simulink model "unifi_GFM_control_demo_single_conv"  (R2020b)
settings: Solver=VariableStepAuto  StartTime=0.0  StopTime=1  MaxStep=1e-3  RelTol=1e-3
InitFcn:
  | % VSC Rating
  | Vnomrms          = 120.0;                                              % [V]
  | Vnom               = Vnomrms*sqrt(2);                             % [V]
  | fnom                = 60.0;                                                % [Hz]
  | Wnom              = 2.0*pi*fnom;                                     % [rad/s]
  | Prated              = 3.0e3;                                               % [W]
  | Qrated             = 1.5e3;                                               % [VAR]
  | Inom               = 2.0*Prated/Vnom/3;                           % [A]
  | Zbase              = Vnom/Inom;                                      % [Ohm]
  | Lbase              = Zbase/Wnom;                                    % [H]
  | 
  | % LCL Filter parameters
  | L1                   = 600e-6;                                            % [H]
  | L2                   = 1e-3;                                                % [H]
  | Cf                    = 22e-6;                                              % [F]
  | R1                   = 20e-3;                                              % [Ohm]
  | R2                   = 20e-3;                                              % [Ohm]
  | Rf                    = 1.5;%20e-3;                                              % [Ohm]
  | 
  | % DC Bus
  | Vdc                  = 380.0;                                               % [V]
  | 
  | % Grid Parameters
  | xOverR             = 20.0;                                                 % [ratio]
  | Lg                    = Lbase*0.2;                                         % [H]
  | Rg                    = Zbase/xOverR*0.2                              % [Ohm]
  | 
  | 
  | % Firmware Parameters
  | IH                     = Inom*1.95;                                        % [A] - HW overcurrent trip limit (instantaneous value)
  | DCL                   = 2.0*Vnom/1.15*0.8;                           % [V]
  | DCH                  = Vdc*1.35;                                          % [V]
  | VGH                  = Vnom*1.5;                                         % [V]
  | 
  | % Droop Parameters
  | maxVolDev         = Vnom*0.05;                                       %[V]
  | maxFreqDev       = Wnom*0.01;                                      %[rad/s]
  | pwDroopCoeff     = maxFreqDev/Prated;                           %[rad/j]
  | qvDroopCoeff      = maxVolDev/Qrated;                            % [V/VAR]
StopFcn:
  | clear functions
libraries: powerlib x27, simulink x4, powerlib_meascontrol x2
settings Model: Creator=mawal  LastModifiedBy=mawal
settings SFSimCC: SimParseCustomCode=off  CustomCodeGlobalsAsFunctionIO=on

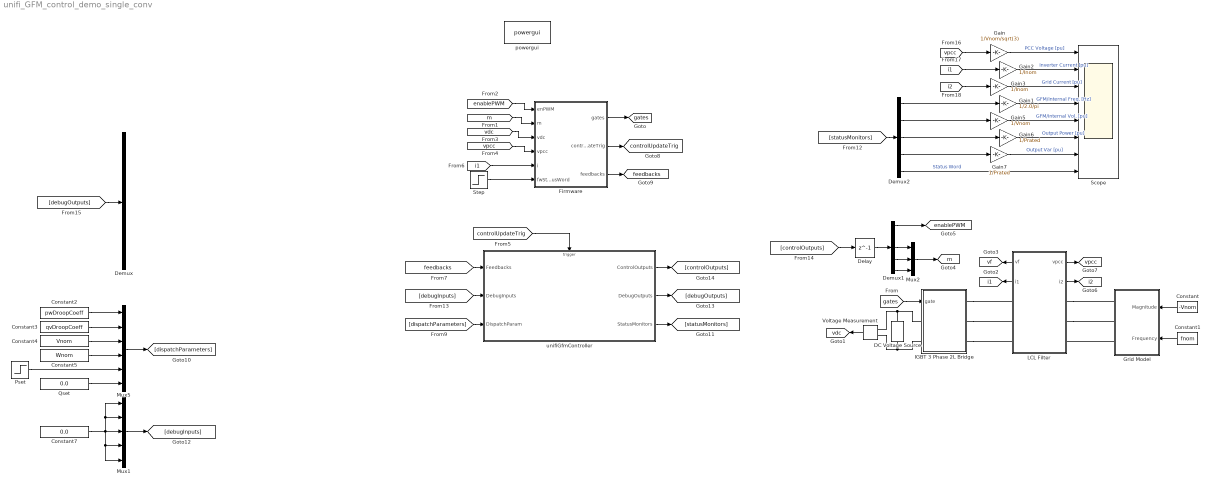
== system unifi_GFM_control_demo_single_conv ==
  Constant : Constant  Value=-Vnom  VectorParams1D=off  SampleTime=-1
  Constant1 : Constant  Value=fnom  VectorParams1D=off  SampleTime=-1
  Constant2 : Constant  Value=pwDroopCoeff
  Constant3 : Constant  Value=qvDroopCoeff
  Constant4 : Constant  Value=Vnom
  Constant5 : Constant  Value=Wnom
  Constant7 : Constant  Value=0.0
  DC Voltage Source : powerlib/Electrical Sources/DC Voltage Source  Amplitude=Vdc  Measurements=None
  Delay : Delay  DelayLength=1
  Demux : Demux  Outputs=10
  Demux1 : Demux  Outputs=5
  Demux2 : Demux  Outputs=5
  Firmware : Subsystem  mask{fsw=50e3, fs=25e3}
      mask prompts: fsw "Switching frequency"; fs "Sampling frequency"
  Gain : Gain  Gain=1/Vnom/sqrt(3)
  Gain1 : Gain  Gain=1/2.0/pi
  Gain2 : Gain  Gain=1/Inom
  Gain3 : Gain  Gain=1/Inom
  Gain5 : Gain  Gain=1/Vnom
  Gain6 : Gain  Gain=1/Prated
  Gain7 : Gain  Gain=1/Prated
  Grid Model : Subsystem
      settings: PortSchema="{\"entries\":[{\"content\":{\"sides\":[{\"content\":{\"connectorIds\":[\"LConn1\",\"LConn2\",\"LConn3\"]},\"type\":\"ConnectorPlacement.EquallySpacedRectSide\",\"uuid\":\"eac9bd49-6506-4418-b391-2d1910dfb123\"},{\"content\":{\"connectorIds\":[\"In1\",\"In2\"],\"side\":\"RIGHT\"},\"type\":\"ConnectorPlacement.EquallySpacedRectSide\",\"uuid\":\"2cf1b579-036f-4489-9916-029144d18b5e\"},{\"content\":{\"connectorIds\":[],\"side\":\"TOP\"},\"type\":\"ConnectorPlacement.EquallySpacedRectSide\",\"uuid\":\"45a6a27e-4276-40c1-8aac-6c9155e67f41\"},{\"content\":{\"connectorIds\":[],\"side\":\"BOTTOM\"},\"type\":\"ConnectorPlacement.EquallySpacedRectSide\",\"uuid\":\"f7ca4a45-1b00-4589-b172-9f3561ecadf3\"},{\"content\":{\"connectorIds\":[],\"side\":\"HIDDEN\"},\"type\":\"ConnectorPlacement.EquallySpacedRectSide\",\"uuid\":\"bf2ee3e7-e909-4e31-bcbb-76e709a5babf\"}]},\"type\":\"ConnectorPlacement.EquallySpacedConnector\",\"uuid\":\"022258a7-3899-4adf-8963-8d60febbe7fe\"}],\"packageUris\":[\"http://schema.mathworks.com/mf0/Connector/R2020b\"],\"version\":\"1.0\"}"
  IGBT 3 Phase 2L Bridge : Subsystem
  LCL Filter : Subsystem
      settings: PortSchema="{\"entries\":[{\"content\":{\"sides\":[{\"content\":{\"connectorIds\":[\"Out3\",\"Out4\",\"LConn1\",\"LConn2\",\"LConn3\"]},\"type\":\"ConnectorPlacement.EquallySpacedRectSide\",\"uuid\":\"3cdc7e29-4b8c-4f58-9b04-3ab9d7132857\"},{\"content\":{\"connectorIds\":[\"Out1\",\"Out2\",\"RConn1\",\"RConn2\",\"RConn3\"],\"side\":\"RIGHT\"},\"type\":\"ConnectorPlacement.EquallySpacedRectSide\",\"uuid\":\"8baa2de2-ce0c-48ae-b26c-b1033ca488ed\"},{\"content\":{\"connectorIds\":[],\"side\":\"TOP\"},\"type\":\"ConnectorPlacement.EquallySpacedRectSide\",\"uuid\":\"794c2f77-a18f-4e85-a713-f814f7818158\"},{\"content\":{\"connectorIds\":[],\"side\":\"HIDDEN\"},\"type\":\"ConnectorPlacement.EquallySpacedRectSide\",\"uuid\":\"a095602e-d5a6-4d5a-a12d-1bc7b692edfa\"}]},\"type\":\"ConnectorPlacement.EquallySpacedConnector\",\"uuid\":\"f071d9f2-7780-45fd-ac97-fd335e4ea6fb\"}],\"packageUris\":[\"http://schema.mathworks.com/mf0/Connector/R2020b\"],\"version\":\"1.0\"}"
  Mux1 : Mux  Inputs=5
  Mux2 : Mux  Inputs=3
  Mux5 : Mux  Inputs=6
  Pset : Step  Time=0.5  Before=0.0  After=Prated  SampleTime=0
  Qset : Constant  Value=0.0
  Scope : Scope  NumInputPorts=8
  Step : Step  Time=0  SampleTime=0
  Voltage Measurement : powerlib/Measurements/Voltage Measurement  PhasorSimulation=off  OutputType=Complex  PSBequivalent=0
  powergui : powerlib/powergui  Priority=1  SimulationMode=Continuous  SampleTime=0.2e-6  frequency=60  Iterations=50  frequencyindice=0  Pbase=100e6  ErrMax=1e-4  UnitsV=kV  UnitsW=MW  buscounter=0  FunctionMessages=off  echomessages=off  EnableUseOfTLC=off  CurrentSourceSwitches=off  DisableSnubberDevices=off  DisableRonSwitches=off  DisableVfSwitches=off  DisplayEquations=off  AutomaticDiscreteSolvers=off  SolverType=Tustin/Backward Euler (TBE)  Interpol=off  ExternalGateDelay=off  methode=off  Ts=100  x0status=blocks  SPID=on  SwTol=0  HookPort=off  NonlinearTolerance=1e-4  nMaxIteration=100  ContinueOnMaxIteration=off  RestoreLinks=warning  ResistiveCurrentMeasurement=off  Frange=[0:2:500]  Ylog=off  Xlog=on  ShowGrid=off  save=off  variable=ZData  structure=0  ZoomFFT=off  StartTime=0.0  cycles=1  DisplayStyle=1  fundamental=60  FreqAxis=off  MaxFrequency=1000  frequencyindicesteady=1  RmsSteady=1  display=off
  unifiGfmController : Subsystem  AncestorBlock=unifi_Sil_Lib/UNIFI SIL Wrapper with Mex Builder  TreatAsAtomicUnit=on
      mask DialogControl importSilTemplate Prompt: Step 1: Import SIL Template
      mask DialogControl importSilTemplate Callback: cbk_import_sil_tem
      mask DialogControl updateInterfaceDim Prompt: Step 2: Update Interface Dimensions (Add/Link custom code prior to Step 2)
      mask DialogControl updateInterfaceDim Callback: cbk_update_interface_dim
      mask DialogControl configMexBuilder Prompt: Step 3: Configure Mex Builder (Disable Library Link to Enable Self-Modification)
      mask DialogControl configMexBuilder Callback: cbk_setup_mex_builder
      mask DialogControl buildMex Prompt: Step 4: Build Mex
      mask DialogControl buildMex Callback: cbk_build_mex
      mask Display: image('$imagefile'); % Use "Edit Image" on toolstrip to change.
  tag scope: controlUpdateTrig=global, enablePWM=global, feedbacks=global, gates=global, i1=global, i2=global, m=global, vdc=global, vf=global, vpcc=global
  wires:
  unifiGfmController/2(DebugOutputs) -> [debugOutputs]
  Firmware/1(gates) -> [gates]
  [gates] -> IGBT 3 Phase 2L Bridge/1(gate)
  Voltage Measurement/1 -> [vdc]
  Constant/1 -> Grid Model/1(Magnitude)
  Constant1/1 -> Grid Model/2(Frequency)
  Demux1/3 -> Mux2/1
  Demux1/4 -> Mux2/2
  Demux1/5 -> Mux2/3
  Mux2/1 -> [m]
  Demux1/1 -> [enablePWM]
  [enablePWM] -> Firmware/1(enPWM)
  [m] -> Firmware/2(m)
  [vdc] -> Firmware/3(vdc)
  [vpcc] -> Firmware/4(vpcc)
  LCL Filter/4(i1) -> [i1]
  LCL Filter/3(vf) -> [vf]
  LCL Filter/2(i2) -> [i2]
  LCL Filter/1(vpcc) -> [vpcc]
  [i1] -> Firmware/5(i)
  Firmware/2(controlUpdateTrig) -> [controlUpdateTrig]
  Firmware/3(feedbacks) -> [feedbacks]
  [feedbacks] -> unifiGfmController/1(Feedbacks)
  Delay/1 -> Demux1/1
  Step/1 -> Firmware/6(fwStatusWord)
  Constant2/1 -> Mux5/1
  Constant3/1 -> Mux5/2
  Constant4/1 -> Mux5/3
  Constant5/1 -> Mux5/4
  Qset/1 -> Mux5/6
  Pset/1 -> Mux5/5
  [dispatchParameters] -> unifiGfmController/3(DispatchParam)
  Mux5/1 -> [dispatchParameters]
  unifiGfmController/3(StatusMonitors) -> [statusMonitors]
  [statusMonitors] -> Demux2/1
  Constant7/1 -> Mux1/2, Mux1/1, Mux1/3, Mux1/5, Mux1/4
  [debugInputs] -> unifiGfmController/2(DebugInputs)
  Mux1/1 -> [debugInputs]
  unifiGfmController/1(ControlOutputs) -> [controlOutputs]
  [controlOutputs] -> Delay/1
  [debugOutputs] -> Demux/1
  Demux2/5 -> Scope/8  "Status Word"
  Demux2/4 -> Gain7/1
  Demux2/3 -> Gain6/1
  Demux2/1 -> Gain1/1
  [vpcc] -> Gain/1
  Gain/1 -> Scope/1  "PCC Voltage [pu]"
  [i1] -> Gain2/1
  Gain2/1 -> Scope/2  "Inverter Current [pu]"
  [i2] -> Gain3/1
  Gain3/1 -> Scope/3  "Grid Current [pu]"
  Gain1/1 -> Scope/4  "GFM/Internal Freq. [Hz]"
  Demux2/2 -> Gain5/1
  Gain5/1 -> Scope/5  "GFM/Internal Vol. [pu]"
  Gain6/1 -> Scope/6  "Output Power [pu]"
  Gain7/1 -> Scope/7  "Output Var [pu]"
  [controlUpdateTrig] -> unifiGfmController/Trigger
  connections:
  IGBT 3 Phase 2L Bridge/RConn2 -- LCL Filter/LConn2
  IGBT 3 Phase 2L Bridge/RConn1 -- LCL Filter/LConn1
  IGBT 3 Phase 2L Bridge/RConn3 -- LCL Filter/LConn3
  DC Voltage Source/RConn1 -- Voltage Measurement/LConn1 -- IGBT 3 Phase 2L Bridge/LConn1
  DC Voltage Source/LConn1 -- Voltage Measurement/LConn2 -- IGBT 3 Phase 2L Bridge/LConn2
  LCL Filter/RConn1 -- Grid Model/LConn1
  LCL Filter/RConn2 -- Grid Model/LConn2
  Grid Model/LConn3 -- LCL Filter/RConn3

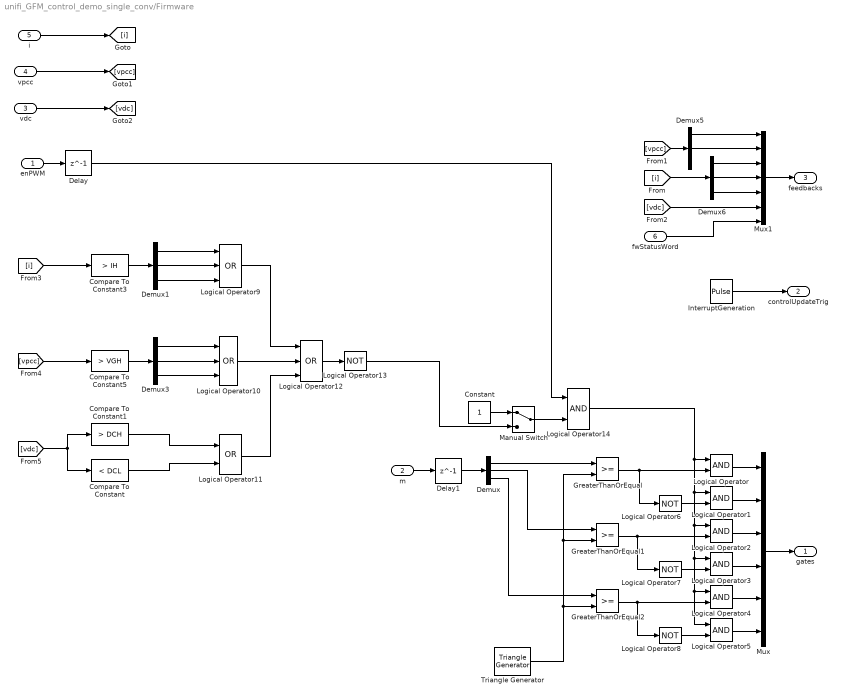
== system unifi_GFM_control_demo_single_conv/Firmware ==
  enPWM : Inport
  m : Inport  Port=2
  vdc : Inport  Port=3
  vpcc : Inport  Port=4
  i : Inport  Port=5
  fwStatusWord : Inport  Port=6
  Compare To Constant : simulink/Logic and Bit Operations/Compare To Constant  relop=<  const=DCL  OutDataTypeStr=boolean
  Compare To Constant1 : simulink/Logic and Bit Operations/Compare To Constant  relop=>  const=DCH  OutDataTypeStr=boolean
  Compare To Constant3 : simulink/Logic and Bit Operations/Compare To Constant  relop=>  const=IH  OutDataTypeStr=boolean
  Compare To Constant5 : simulink/Logic and Bit Operations/Compare To Constant  relop=>  const=VGH  OutDataTypeStr=boolean
  Constant : Constant
  Delay : Delay  DelayLength=1
  Delay1 : Delay  DelayLength=1
  Demux{,1,3,5..6} (5 alike) : Demux  Outputs=3
  GreaterThanOrEqual : RelationalOperator  OutDataTypeStr=boolean  RndMeth=Simplest
  GreaterThanOrEqual1 : RelationalOperator  OutDataTypeStr=boolean  RndMeth=Simplest
  GreaterThanOrEqual2 : RelationalOperator  OutDataTypeStr=boolean  RndMeth=Simplest
  InterruptGeneration : DiscretePulseGenerator  PulseType=Time based  Period=1/fs  PulseWidth=50
  Logical Operator{,1..5,14} (7 alike) : Logic  AllPortsSameDT=off  OutDataTypeStr=boolean
  Logical Operator10 : Logic  Operator=OR  Inputs=3  AllPortsSameDT=off  OutDataTypeStr=boolean
  Logical Operator11 : Logic  Operator=OR  AllPortsSameDT=off  OutDataTypeStr=boolean
  Logical Operator12 : Logic  Operator=OR  Inputs=3  AllPortsSameDT=off  OutDataTypeStr=boolean
  Logical Operator13 : Logic  Operator=NOT  Inputs=3  AllPortsSameDT=off  OutDataTypeStr=boolean
  Logical Operator6 : Logic  Operator=NOT  AllPortsSameDT=off  OutDataTypeStr=boolean
  Logical Operator7 : Logic  Operator=NOT  AllPortsSameDT=off  OutDataTypeStr=boolean
  Logical Operator8 : Logic  Operator=NOT  AllPortsSameDT=off  OutDataTypeStr=boolean
  Logical Operator9 : Logic  Operator=OR  Inputs=3  AllPortsSameDT=off  OutDataTypeStr=boolean
  Manual Switch : ManualSwitch
  Mux : Mux  Inputs=6
  Mux1 : Mux  Inputs=7
  Triangle Generator : powerlib_meascontrol/Pulse & Signal Generators/Triangle Generator  Freq=fsw  Phase=0  Ts=0
  gates : Outport
  controlUpdateTrig : Outport  Port=2
  feedbacks : Outport  Port=3
  wires:
  Triangle Generator/1 -> GreaterThanOrEqual2/2, GreaterThanOrEqual1/2, GreaterThanOrEqual/2
  Logical Operator/1 -> Mux/1
  Logical Operator1/1 -> Mux/2
  Logical Operator2/1 -> Mux/3
  Logical Operator3/1 -> Mux/4
  Logical Operator4/1 -> Mux/5
  Logical Operator5/1 -> Mux/6
  GreaterThanOrEqual/1 -> Logical Operator/2, Logical Operator6/1
  Logical Operator6/1 -> Logical Operator1/2
  Logical Operator7/1 -> Logical Operator3/2
  GreaterThanOrEqual1/1 -> Logical Operator7/1, Logical Operator2/2
  GreaterThanOrEqual2/1 -> Logical Operator8/1, Logical Operator4/2
  Logical Operator8/1 -> Logical Operator5/2
  m/1 -> Delay1/1
  Demux/1 -> GreaterThanOrEqual/1
  Demux/2 -> GreaterThanOrEqual1/1
  Demux/3 -> GreaterThanOrEqual2/1
  Compare To Constant3/1 -> Demux1/1
  Demux1/1 -> Logical Operator9/1
  Demux1/2 -> Logical Operator9/2
  Demux1/3 -> Logical Operator9/3
  Compare To Constant5/1 -> Demux3/1
  Demux3/1 -> Logical Operator10/1
  Demux3/2 -> Logical Operator10/2
  Demux3/3 -> Logical Operator10/3
  Compare To Constant1/1 -> Logical Operator11/1
  Compare To Constant/1 -> Logical Operator11/2
  Logical Operator10/1 -> Logical Operator12/2
  Logical Operator9/1 -> Logical Operator12/1
  Logical Operator11/1 -> Logical Operator12/3
  Logical Operator12/1 -> Logical Operator13/1
  Mux/1 -> gates/1
  enPWM/1 -> Delay/1
  Logical Operator14/1 -> Logical Operator5/1, Logical Operator4/1, Logical Operator3/1, Logical Operator2/1, Logical Operator1/1, Logical Operator/1
  Manual Switch/1 -> Logical Operator14/2
  Logical Operator13/1 -> Manual Switch/2
  Constant/1 -> Manual Switch/1
  InterruptGeneration/1 -> controlUpdateTrig/1
  Demux6/1 -> Mux1/3
  Demux5/2 -> Mux1/2
  Demux6/2 -> Mux1/4
  Demux6/3 -> Mux1/5
  Demux5/1 -> Mux1/1
  i/1 -> [i]
  vpcc/1 -> [vpcc]
  vdc/1 -> [vdc]
  [i] -> Demux6/1
  [vpcc] -> Demux5/1
  [vdc] -> Mux1/6
  [vpcc] -> Compare To Constant5/1
  [i] -> Compare To Constant3/1
  [vdc] -> Compare To Constant1/1, Compare To Constant/1
  fwStatusWord/1 -> Mux1/7
  Mux1/1 -> feedbacks/1
  Delay/1 -> Logical Operator14/1
  Delay1/1 -> Demux/1

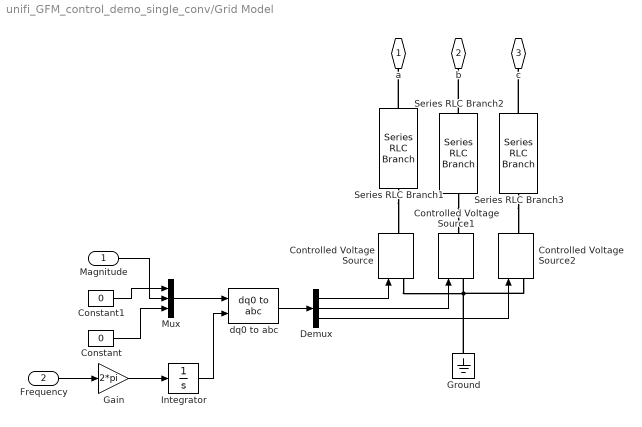
== system unifi_GFM_control_demo_single_conv/Grid Model ==
  Magnitude : Inport
  Frequency : Inport  Port=2
  Constant : Constant  Value=0
  Constant1 : Constant  Value=0
  Controlled Voltage Source : powerlib/Electrical Sources/Controlled Voltage Source  Initialize=on  Source_Type=AC  Amplitude=0  Phase=0  Frequency=0  Measurements=None
  Controlled Voltage Source1 : powerlib/Electrical Sources/Controlled Voltage Source  Initialize=on  Source_Type=AC  Amplitude=0  Phase=0  Frequency=0  Measurements=None
  Controlled Voltage Source2 : powerlib/Electrical Sources/Controlled Voltage Source  Initialize=on  Source_Type=AC  Amplitude=0  Phase=0  Frequency=0  Measurements=None
  Demux : Demux  Outputs=3
  Gain : Gain  Gain=2*pi
  Ground : powerlib/Elements/Ground  LConnTagsString=a
  Integrator : Integrator  InitialCondition=pi/3  WrapState=on
  Mux : Mux  Inputs=3
  Series RLC Branch1 : powerlib/Elements/Series RLC Branch  LConnTagsString=__new0  RConnTagsString=__new0  BranchType=RL  Resistance=Rg  Inductance=Lg  SetiL0=off  InitialCurrent=0  Capacitance=1e-6  Setx0=off  InitialVoltage=0  Measurements=None
  Series RLC Branch2 : powerlib/Elements/Series RLC Branch  LConnTagsString=__new0  RConnTagsString=__new0  BranchType=RL  Resistance=Rg  Inductance=Lg  SetiL0=off  InitialCurrent=0  Capacitance=1e-6  Setx0=off  InitialVoltage=0  Measurements=None
  Series RLC Branch3 : powerlib/Elements/Series RLC Branch  LConnTagsString=__new0  RConnTagsString=__new0  BranchType=RL  Resistance=Rg  Inductance=Lg  SetiL0=off  InitialCurrent=0  Capacitance=1e-6  Setx0=off  InitialVoltage=0  Measurements=None
  dq0 to abc : powerlib_meascontrol/Transformations/dq0 to abc  Alignment=90 degrees behind phase A axis
  a : PMIOPort  Side=Left
  b : PMIOPort  Port=2  Side=Left
  c : PMIOPort  Port=3  Side=Left
  wires:
  Gain/1 -> Integrator/1
  Constant/1 -> Mux/3
  Frequency/1 -> Gain/1
  Mux/1 -> dq0 to abc/1
  Integrator/1 -> dq0 to abc/2
  dq0 to abc/1 -> Demux/1
  Demux/1 -> Controlled Voltage Source/1
  Demux/2 -> Controlled Voltage Source1/1
  Demux/3 -> Controlled Voltage Source2/1
  Constant1/1 -> Mux/1
  Magnitude/1 -> Mux/2
  connections:
  Controlled Voltage Source/LConn1 -- Ground/LConn1 -- Controlled Voltage Source2/LConn1 -- Controlled Voltage Source1/LConn1
  Series RLC Branch1/RConn1 -- Controlled Voltage Source/RConn1
  Series RLC Branch1/LConn1 -- a/RConn1
  Series RLC Branch2/LConn1 -- b/RConn1
  Series RLC Branch2/RConn1 -- Controlled Voltage Source1/RConn1
  Series RLC Branch3/LConn1 -- c/RConn1
  Series RLC Branch3/RConn1 -- Controlled Voltage Source2/RConn1

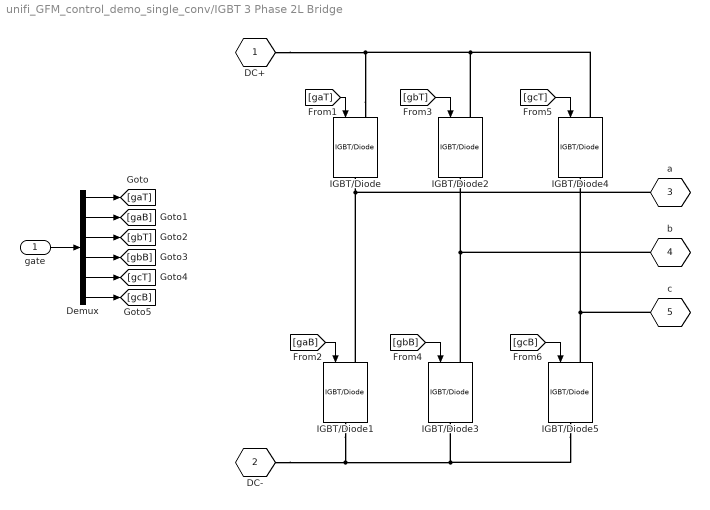
== system unifi_GFM_control_demo_single_conv/IGBT 3 Phase 2L Bridge ==
  gate : Inport
  Demux : Demux  Outputs=6
  IGBT/Diode{,1..5} (6 alike) : powerlib/Power Electronics/IGBT//Diode  Ron=1e-3  Rs=1e5  Cs=inf  Measurements=off
  DC+ : PMIOPort  Tag=PMCPort  Side=Left
  DC- : PMIOPort  Tag=PMCPort  Port=2  Side=Left
  a : PMIOPort  Tag=PMCPort  Port=3  Side=Right
  b : PMIOPort  Tag=PMCPort  Port=4  Side=Right
  c : PMIOPort  Tag=PMCPort  Port=5  Side=Right
  wires:
  [gaT] -> IGBT/Diode/1
  [gaB] -> IGBT/Diode1/1
  [gbT] -> IGBT/Diode2/1
  [gbB] -> IGBT/Diode3/1
  [gcT] -> IGBT/Diode4/1
  [gcB] -> IGBT/Diode5/1
  gate/1 -> Demux/1
  Demux/1 -> [gaT]
  Demux/2 -> [gaB]
  Demux/3 -> [gbT]
  Demux/4 -> [gbB]
  Demux/5 -> [gcT]
  Demux/6 -> [gcB]
  connections:
  IGBT/Diode3/LConn1 -- b/RConn1 -- IGBT/Diode2/RConn1
  IGBT/Diode/LConn1 -- DC+/RConn1 -- IGBT/Diode4/LConn1 -- IGBT/Diode2/LConn1
  IGBT/Diode5/LConn1 -- c/RConn1 -- IGBT/Diode4/RConn1
  IGBT/Diode1/RConn1 -- DC-/RConn1 -- IGBT/Diode3/RConn1 -- IGBT/Diode5/RConn1
  IGBT/Diode1/LConn1 -- a/RConn1 -- IGBT/Diode/RConn1

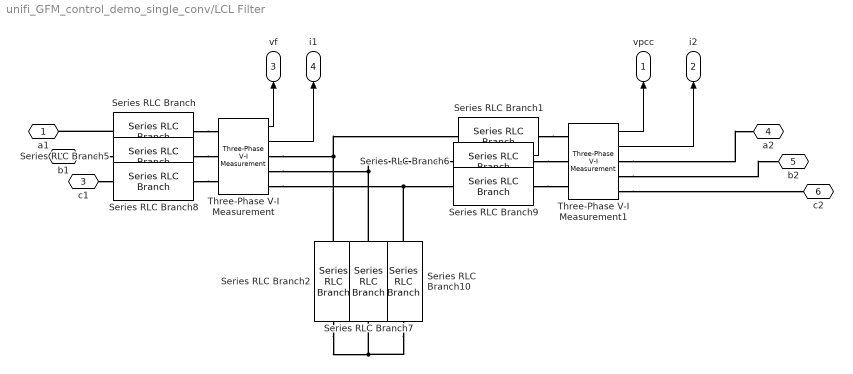
== system unifi_GFM_control_demo_single_conv/LCL Filter ==
  Series RLC Branch : powerlib/Elements/Series RLC Branch  LConnTagsString=__new0  RConnTagsString=__new0  BranchType=RL  Resistance=R1  Inductance=L1  SetiL0=off  InitialCurrent=0  Capacitance=1e-6  Setx0=off  InitialVoltage=0  Measurements=None
  Series RLC Branch1 : powerlib/Elements/Series RLC Branch  LConnTagsString=__new0  RConnTagsString=__new0  BranchType=RL  Resistance=R2  Inductance=L2  SetiL0=off  InitialCurrent=0  Capacitance=1e-6  Setx0=off  InitialVoltage=0  Measurements=None
  Series RLC Branch10 : powerlib/Elements/Series RLC Branch  LConnTagsString=__new0  RConnTagsString=__new0  BranchType=RC  Resistance=Rf  Inductance=L1  SetiL0=off  InitialCurrent=0  Capacitance=Cf  Setx0=off  InitialVoltage=0  Measurements=None
  Series RLC Branch2 : powerlib/Elements/Series RLC Branch  LConnTagsString=__new0  RConnTagsString=__new0  BranchType=RC  Resistance=Rf  Inductance=L1  SetiL0=off  InitialCurrent=0  Capacitance=Cf  Setx0=off  InitialVoltage=0  Measurements=None
  Series RLC Branch5 : powerlib/Elements/Series RLC Branch  LConnTagsString=__new0  RConnTagsString=__new0  BranchType=RL  Resistance=R1  Inductance=L1  SetiL0=off  InitialCurrent=0  Capacitance=1e-6  Setx0=off  InitialVoltage=0  Measurements=None
  Series RLC Branch6 : powerlib/Elements/Series RLC Branch  LConnTagsString=__new0  RConnTagsString=__new0  BranchType=RL  Resistance=R2  Inductance=L2  SetiL0=off  InitialCurrent=0  Capacitance=1e-6  Setx0=off  InitialVoltage=0  Measurements=None
  Series RLC Branch7 : powerlib/Elements/Series RLC Branch  LConnTagsString=__new0  RConnTagsString=__new0  BranchType=RC  Resistance=Rf  Inductance=L1  SetiL0=off  InitialCurrent=0  Capacitance=Cf  Setx0=off  InitialVoltage=0  Measurements=None
  Series RLC Branch8 : powerlib/Elements/Series RLC Branch  LConnTagsString=__new0  RConnTagsString=__new0  BranchType=RL  Resistance=R1  Inductance=L1  SetiL0=off  InitialCurrent=0  Capacitance=1e-6  Setx0=off  InitialVoltage=0  Measurements=None
  Series RLC Branch9 : powerlib/Elements/Series RLC Branch  LConnTagsString=__new0  RConnTagsString=__new0  BranchType=RL  Resistance=R2  Inductance=L2  SetiL0=off  InitialCurrent=0  Capacitance=1e-6  Setx0=off  InitialVoltage=0  Measurements=None
  Three-Phase V-I Measurement : powerlib/Measurements/Three-Phase V-I Measurement  VoltageMeasurement=phase-to-phase  SetLabelV=off  LabelV=Vabc  Vpu=off  VpuLL=off  CurrentMeasurement=yes  SetLabelI=off  LabelI=Iabc  Ipu=off  Pbase=100e6  Vbase=500e3  OutputType=Complex  PhasorSimulation=off  PSBequivalent=0
  Three-Phase V-I Measurement1 : powerlib/Measurements/Three-Phase V-I Measurement  VoltageMeasurement=phase-to-phase  SetLabelV=off  LabelV=Vabc  Vpu=off  VpuLL=off  CurrentMeasurement=yes  SetLabelI=off  LabelI=Iabc  Ipu=off  Pbase=100e6  Vbase=500e3  OutputType=Complex  PhasorSimulation=off  PSBequivalent=0
  a1 : PMIOPort  Side=Left
  b1 : PMIOPort  Port=2  Side=Left
  c1 : PMIOPort  Port=3  Side=Left
  a2 : PMIOPort  Port=4  Side=Right
  b2 : PMIOPort  Port=5  Side=Right
  c2 : PMIOPort  Port=6  Side=Right
  vpcc : Outport
  i2 : Outport  Port=2
  vf : Outport  Port=3
  i1 : Outport  Port=4
  wires:
  Three-Phase V-I Measurement/2 -> i1/1
  Three-Phase V-I Measurement/1 -> vf/1
  Three-Phase V-I Measurement1/2 -> i2/1
  Three-Phase V-I Measurement1/1 -> vpcc/1
  connections:
  Series RLC Branch2/LConn1 -- Series RLC Branch1/LConn1 -- Three-Phase V-I Measurement/RConn1
  Series RLC Branch/LConn1 -- a1/RConn1
  Series RLC Branch7/LConn1 -- Series RLC Branch6/LConn1 -- Three-Phase V-I Measurement/RConn2
  Series RLC Branch10/LConn1 -- Series RLC Branch9/LConn1 -- Three-Phase V-I Measurement/RConn3
  Series RLC Branch/RConn1 -- Three-Phase V-I Measurement/LConn1
  Series RLC Branch5/RConn1 -- Three-Phase V-I Measurement/LConn2
  Series RLC Branch8/RConn1 -- Three-Phase V-I Measurement/LConn3
  Series RLC Branch2/RConn1 -- Series RLC Branch10/RConn1 -- Series RLC Branch7/RConn1
  b1/RConn1 -- Series RLC Branch5/LConn1
  c1/RConn1 -- Series RLC Branch8/LConn1
  Series RLC Branch1/RConn1 -- Three-Phase V-I Measurement1/LConn1
  Series RLC Branch6/RConn1 -- Three-Phase V-I Measurement1/LConn2
  Series RLC Branch9/RConn1 -- Three-Phase V-I Measurement1/LConn3
  Three-Phase V-I Measurement1/RConn1 -- a2/RConn1
  Three-Phase V-I Measurement1/RConn2 -- b2/RConn1
  Three-Phase V-I Measurement1/RConn3 -- c2/RConn1

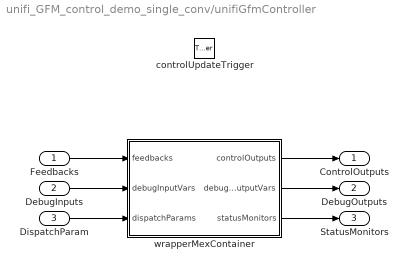
== system unifi_GFM_control_demo_single_conv/unifiGfmController ==
  Feedbacks : Inport
  DebugInputs : Inport  Port=2
  DispatchParam : Inport  Port=3
  controlUpdateTrigger : TriggerPort  VariantControl=Variant
  wrapperMexContainer : MATLAB Function  TreatAsAtomicUnit=on
  ControlOutputs : Outport
  DebugOutputs : Outport  Port=2
  StatusMonitors : Outport  Port=3
  wires:
  wrapperMexContainer/3(statusMonitors) -> StatusMonitors/1
  wrapperMexContainer/2(debugOutputVars) -> DebugOutputs/1
  wrapperMexContainer/1(controlOutputs) -> ControlOutputs/1
  DispatchParam/1 -> wrapperMexContainer/3(dispatchParams)
  DebugInputs/1 -> wrapperMexContainer/2(debugInputVars)
  Feedbacks/1 -> wrapperMexContainer/1(feedbacks)

== matlab function unifi_GFM_control_demo_single_conv/unifiGfmController/wrapperMexContainer ==
  data: feedbacks input; controlOutputs output; debugInputVars input; dispatchParams input; debugOutputVars output; statusMonitors output
function [controlOutputs, debugOutputVars, statusMonitors] = runWrapperMex(feedbacks, debugInputVars, dispatchParams)
numberOfDebugOutVars = 10;
numberOfControlOutVars = 5;
numberOfStatusMonitors = 5;

controlOutputs  = zeros(numberOfControlOutVars, 1);
debugOutputVars = zeros(numberOfDebugOutVars, 1);
statusMonitors  = zeros(numberOfStatusMonitors, 1);
coder.extrinsic('unifiGfmController_mex');

[vcontrolOutputs, vdebugOutputVars, vstatusMonitors] = ...
    unifiGfmController_mex(feedbacks,debugInputVars, dispatchParams);

controlOutputs  = double(vcontrolOutputs);
debugOutputVars = double(vdebugOutputVars);
statusMonitors  = double(vstatusMonitors);
end
